simulink model "blockDiag"  (R2021a)
settings: Solver=VariableStepAuto  StartTime=0.0  StopTime=250  RelTol=1e-3
values from neighbouring files (symbols this model uses):
  GB = 110    [param.m]
  p1 = 0.028    [param.m]
  p2 = 0.025    [param.m]
  p3 = 0.00013    [param.m]
  p4 = 5/54    (= 0.0925925925926)    [param.m]
  VL = 120    [param.m]
settings Model: Creator=gabri  LastModifiedBy=gabri

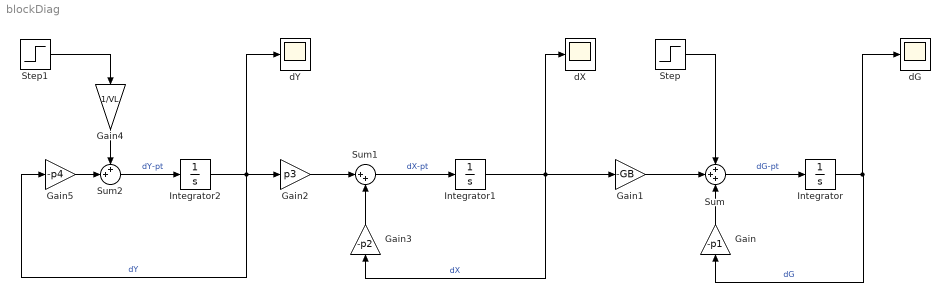
== system blockDiag ==
  Gain : Gain  Gain=-p1
  Gain1 : Gain  Gain=-GB
  Gain2 : Gain  Gain=p3
  Gain3 : Gain  Gain=-p2
  Gain4 : Gain  Gain=1/VL
  Gain5 : Gain  Gain=-p4
  Integrator : Integrator
  Integrator1 : Integrator
  Integrator2 : Integrator
  Step : Step  SampleTime=0
  Step1 : Step  SampleTime=0
  Sum : Sum  Inputs=+++
  Sum1 : Sum  Inputs=|++
  Sum2 : Sum  Inputs=++|
  dG : Scope
  dX : Scope
  dY : Scope
  wires:
  Gain1/1 -> Sum/2
  Step/1 -> Sum/1
  Gain/1 -> Sum/3
  Sum/1 -> Integrator/1  "dG-pt"
  Integrator/1 -> dG/1, Gain/1  "dG"
  Gain2/1 -> Sum1/1
  Gain3/1 -> Sum1/2
  Sum1/1 -> Integrator1/1  "dX-pt"
  Integrator1/1 -> dX/1, Gain1/1, Gain3/1  "dX"
  Step1/1 -> Gain4/1
  Gain4/1 -> Sum2/1
  Gain5/1 -> Sum2/2
  Sum2/1 -> Integrator2/1  "dY-pt"
  Integrator2/1 -> dY/1, Gain2/1, Gain5/1  "dY"
